simulink model "AFCS_MODEL1"  (R2020b)
settings: Solver=ode4  StartTime=0.0  StopTime=inf  FixedStep=0.005  RelTol=1e-3  EnableMultiTasking=on
values from neighbouring files (symbols this model uses):
  mulh0 = [Lat0;Lon0;Alt0]    [Initial.m]
  routedata_NEH = zeros(3,30)    [Initial.m]
  routeNum = 17    [Initial.m]
libraries: slrealtimeutilitieslib x2, dspnetwork x2, aerolibanimutils x1, simulink x1
settings Model: Creator=Unicorn  LastModifiedBy=chenjiaqing
settings DataIOCC: ReturnWorkspaceOutputs=off
settings OptimizationCC: LifeSpan=inf
settings DebuggingCC: SFUnexpectedBacktrackingDiag=warning  SFNoUnconditionalDefaultTransitionDiag=warning  ArithmeticOperatorsInVariantConditions=warning
settings SFSimCC: SimUseLocalCustomCode=off  CustomCodeUndefinedFunction=UseInterfaceOnly
settings RTWCC: RTWUseLocalCustomCode=off
settings CodeAppCC: StateflowObjectComments=on
settings GRTTargetCC: TargetLangStandard=C89/C90 (ANSI)
settings ConfigComp: CovMetricSettings=dw  CovSaveCumulativeToWorkspaceVar=on  CovSaveSingleToWorkspaceVar=on  CovExternalEMLEnable=off

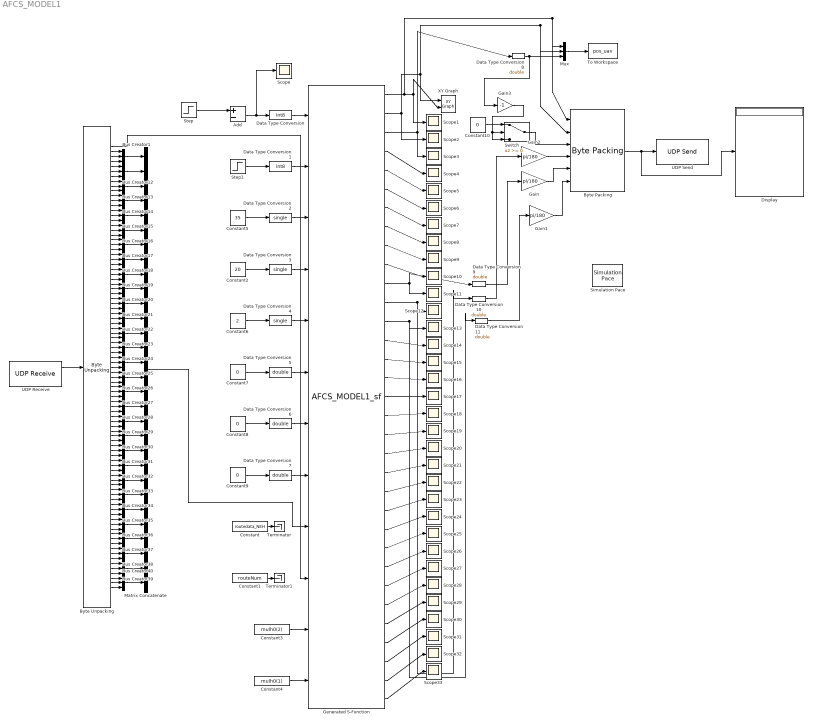
== system AFCS_MODEL1 ==
  Add : Sum  Inputs=+-
  Bus Creator{1,12..40} (30 alike) : BusCreator  Inputs=3
  Byte Packing : slrealtimeutilitieslib/Byte Packing  MaskPackedDataType=double  MaskUnpackedDataTypes={'double','double','double','double','double','double'}  MaskAlignment=8
  Byte Unpacking : slrealtimeutilitieslib/Byte Unpacking  MaskUnpackedDataTypes={'double','double','double','double','double','double','double','double','double','double','double','double','double','double','double','double','double','double','double','double','double','double','double','double','double','double','double','double','double','double','double','double','double','double','double','double','double','double','double','double','double','double','double','double','double','double','double','double','double','double','double','double','double','double','double','double','double','double','double','double','double','double','double','double','double','double','double','double','double','double','double','double','double','double','double','double','double','double','double','double','double','double','double','double','double','double','double','double','double','double','double'}  MaskUnpackedDataSizes={[1],[1],[1],[1],[1],[1],[1],[1],[1],[1],[1],[1],[1],[1],[1],[1],[1],[1],[1],[1],[1],[1],[1],[1],[1],[1],[1],[1],[1],[1],[1],[1],[1],[1],[1],[1],[1],[1],[1],[1],[1],[1],[1],[1],[1],[1],[1],[1],[1],[1],[1],[1],[1],[1],[1],[1],[1],[1],[1],[1],[1],[1],[1],[1],[1],[1],[1],[1],[1],[1],[1],[1],[1],[1],[1],[1],[1],[1],[1],[1],[1],[1],[1],[1],[1],[1],[1],[1],[1],[1],[1]}  MaskAlignment=1
      settings: SourceProductBaseCode=XP
  Constant : Constant  Value=routedata_NEH
  Constant1 : Constant  Value=routeNum
  Constant{7..10} (4 alike) : Constant  Value=0
  Constant2 : Constant  Value=20
  Constant3 : Constant  Value=mulh0(2)
  Constant4 : Constant  Value=mulh0(1)
  Constant5 : Constant  Value=35
  Constant6 : Constant  Value=2
  Data Type Conversion : DataTypeConversion  OutDataTypeStr=int8
  Data Type Conversion1 : DataTypeConversion  OutDataTypeStr=int8
  Data Type Conversion{5..11} (7 alike) : DataTypeConversion  OutDataTypeStr=double
  Data Type Conversion2 : DataTypeConversion  OutDataTypeStr=single
  Data Type Conversion3 : DataTypeConversion  OutDataTypeStr=single
  Data Type Conversion4 : DataTypeConversion  OutDataTypeStr=single
  Display : Display
  Gain : Gain  Gain=pi/180
  Gain1 : Gain  Gain=pi/180
  Gain2 : Gain  Gain=pi/180
  Gain3 : Gain  Gain=-1
  Generated S-Function : S-Function  FunctionName=AFCS_MODEL1_sf  SFunctionModules=""  SFunctionDeploymentMode=off  EnableBusSupport=off  SFcnStateName=DWORK0,DWORK1,DWORK146,DWORK147,DWORK148,DWORK149,DWORK150,DWORK151,DWORK152,DWORK153,DWORK154,DWORK155,DWORK156,DWORK157,DWORK158,DWORK159,DWORK160,DWORK161,DWORK162,DWORK163,DWORK164,DWORK165,DWORK166,DWORK167,DWORK168,DWORK169,DWORK170,DWORK171,DWORK172,DWORK173,DWORK174,DWORK175,DWORK176,DWORK177,DWORK178,DWORK179,DWORK180,DWORK181,DWORK182,DWORK183,DWORK184,DWORK185,DWORK186,DWORK187,DWORK188,DWORK189,DWORK190,DWORK191,DWORK192,DWORK193,DWORK194,DWORK195,DWORK196,DWORK197,DWORK198,DWORK199,DWORK200,DWORK201,DWORK202,DWORK203,DWORK204,DWORK205,DWORK206,DWORK207,DWORK208,DWORK209,DWORK210,DWORK211,DWORK212,DWORK213,DWORK214,DWORK215,DWORK216,DWORK217,DWORK218,DWORK219,DWORK220,DWORK221,DWORK222,DWORK223,DWORK224,DWORK225,DWORK226,DWORK227,DWORK228,DWORK229,DWORK230,DWORK231,DWORK232,DWORK233,DWORK234,DWORK235,DWORK236,DWORK237,DWORK238,DWORK239,DWORK240,DWORK241,DWORK242,DWORK243,DWORK244,DWORK245,DWORK246,DWORK247,DWORK248,DWORK249,DWORK250,DWORK251,DWORK252,DWORK253,DWORK254,DWORK255,DWORK256,DWORK257,DWORK258,DWORK259,DWORK260,DWORK261,DWORK262,DWORK263,DWORK264,DWORK265,DWORK266,DWORK267,DWORK268,DWORK269,DWORK352,DWORK353,DWORK354,DWORK355,DWORK356,DWORK357,DWORK358,DWORK359,DWORK360,DWORK361,DWORK362,DWORK363,DWORK364,DWORK365,DWORK366,DWORK367,DWORK368,DWORK369,DWORK370,DWORK371,DWORK372,DWORK373,DWORK374,DWORK375,DWORK376,DWORK377,DWORK378,DWORK379,DWORK380,DWORK381,DWORK382,DWORK383,DWORK384,DWORK385,DWORK386,DWORK387,DWORK388,DWORK389,DWORK390,DWORK391,DWORK392,DWORK393,DWORK394,DWORK395,DWORK396,DWORK397,DWORK398,DWORK399,DWORK400,DWORK401,DWORK402,DWORK403,DWORK404,DWORK405,DWORK406,DWORK407,DWORK408,DWORK409,DWORK410,DWORK411,DWORK412,DWORK413,DWORK414,DWORK415,DWORK416,DWORK417,DWORK418,DWORK419,DWORK420,DWORK421,DWORK422,DWORK423,DWORK424,DWORK425,DWORK426,DWORK427,DWORK428,DWORK429,DWORK430,DWORK431,DWORK432,DWORK433,DWORK434,DWORK435,DWORK436,DWORK437,DWORK438,DWORK439,DWORK440,DWORK441,DWORK442,DWORK443,DWORK444,DWORK445,DWORK446,DWORK447,DWORK448,DWORK449,DWORK450,DWORK451,DWORK452,DWORK453,DWORK454,DWORK455,DWORK456,DWORK457,DWORK458,DWORK459,DWORK460,DWORK461,DWORK462,DWORK463,DWORK464,DWORK465,DWORK466,DWORK467,DWORK468,DWORK469,DWORK470,DWORK471,DWORK472,DWORK473,DWORK474,DWORK475,DWORK476,DWORK477,DWORK478,DWORK479,DWORK480,DWORK481,DWORK482,DWORK483,DWORK484,DWORK485,DWORK486,DWORK487,DWORK488,DWORK489,DWORK490,DWORK491,DWORK492,DWORK493,DWORK494,DWORK495,DWORK496,DWORK497,DWORK498,DWORK499,DWORK500,DWORK501,DWORK502,DWORK503  mask{rtw_sf_name=AFCS_MODEL1_sf, showVar=off}
      mask prompts: rtw_sf_name "Simulink:masks:GenSFuncName_MP"; showVar "Simulink:masks:GenSFuncShowModuleList_MP"
      mask help: Simulink:masks:GenSFuncDesc_MD
      mask init:
      | displist = '';
      | if ~strcmp(get_param(gcb, 'FunctionName'), rtw_sf_name);
      |   set_param(gcb, 'FunctionName', rtw_sf_name);
      | end
      | % Check if we are generating code
      | rtw_mode = false;
      | if strcmpi(get_param(bdroot(gcb),'SimulationStatus'),'Initializing')
      | 	rtw_mode = strcmpi(get_param(bdroot(gcb),'BuildingRTWCode'),'on') && ...
      | 		~strcmpi(get_param(bdroot(gcb),'TargetStyle'),'SimulationTarget');
      | end
      | if showVar || rtw_mode
      | 	if exist('rtwsfunc') == 2 | exist('rtwsfunc') == 6
      | 		tmplist = rtwsfunc(rtw_sf_name,gcb);
      | 		tmplist = DAStudio.message('Simulink:masks:GenSFuncListOfModules_IC', tmplist);
      | 	elseif showVar
      | 		tmplist1 = DAStudio.message('Simulink:masks:GenSFuncListOfModules_IC', '');
      |         tmplist2 = DAStudio.message('Simulink:masks:GenSFuncNotLicensed_IC');
      |         tmplist = [tmplist1 tmplist2];
      |  	end
      | end
      | if showVar
      |   displist = tmplist;
      | end
      settings: SFcnIsStateOwnerBlock=on
      settings: CopyFcn=|
      | if ~strcmp(get_param(gcb,'Linkstatus'),'none') && ...
      | ~strcmp(get_param(gcb,'Linkstatus'),'implicit')
      |   set_param(gcb,'LinkStatus','none');
      | end
      mask Help: eval('feval(''rtwprivate'',''rtwhelpview'',''rtw_sfcn_block'')');
      mask Display:
      | port_label('input',1,'YD_MODE');
      | port_label('input',2,'AT_MODE');
      | port_label('input',3,'DV');
      | port_label('input',4,'CMD_PhiC');
      | port_label('input',5,'CMD_HdotC');
      | port_label('input',6,'Vx_wind');
      | port_label('input',7,'Vy_wind');
      | port_label('input',8,'Vz_wind');
      | port_label('input',9,'routedata_NEH');
      | port_label('input',10,'piontNum');
      | port_label('input',11,'lon0');
      | port_label('input',12,'lat0');
      | port_label('output',1,'X');
      | port_label('output',2,'Y');
      | port_label('output',3,'Hp');
      | port_label('output',4,'HBC');
      | port_label('output',5,'Hg');
      | port_label('output',6,'Vx');
      | port_label('output',7,'Vy');
      | port_label('output',8,'Vh');
      | port_label('output',9,'Alpha');
      | port_label('output',10,'Beta');
      | port_label('output',11,'Theta');
      | port_label('output',12,'Phi');
      | port_label('output',13,'Psi');
      | port_label('output',14,'TRK');
      | port_label('output',15,'p');
      | port_label('output',16,'q');
      | port_label('output',17,'r');
      | port_label('output',18,'Ax');
      | port_label('output',19,'Ay');
      | port_label('output',20,'Az');
      | port_label('output',21,'PLA_L');
      | port_label('output',22,'PLA_R');
      | port_label('output',23,'N2_L');
      | port_label('output',24,'N2_R');
      | port_label('output',25,'De_L');
      | port_label('output',26,'De_R');
      | port_label('output',27,'Da_L');
      | port_label('output',28,'Da_R');
      | port_label('output',29,'Dr');
      | port_label('output',30,'VIAS');
      | port_label('output',31,'VTAS');
      | port_label('output',32,'VG');
      | port_label('output',33,'Flyphase');
  Matrix Concatenate : Concatenate  NumInputs=30  Mode=Multidimensional array  ConcatenateDimension=2
  Mux : Mux  Inputs=3
  Scope{,1..33} (34 alike) : Scope
  Simulation Pace : aerolibanimutils/Simulation Pace  SimulationPace=1  SleepMode=MATLAB Thread  OutputPaceError=off  SampleTime=-1
  Step : Step  Time=100  After=0  SampleTime=0
  Step1 : Step  Time=60  SampleTime=0
  Switch : Switch
  Terminator : Terminator
  Terminator1 : Terminator
  To Workspace : ToWorkspace  VariableName=pos_uav  SampleTime=-1
  UDP Receive : dspnetwork/UDP Receive  localURL='0.0.0.0'  localPort=udp_receive0  remoteURL='127.0.0.1'  remotePort=-1  recvBufferSize=91  dims=91  signalDatatype=double  isComplex=off  isVarSize=off  showBlockingTime=off  blockingTime=0  sampletime=-1  blockPlatform=[]
  UDP Send : dspnetwork/UDP Send  remoteURL='127.0.0.1'  remotePort=udp_send0  localURL='0.0.0.0'  localPortSource=Automatically determine  localPort=25000  sendBufferSize=1  sampletime=-1  blockPlatform=[]  separateLengthPort=0
  XY Graph : simulink/Sinks/XY Graph  xmin=-3000  xmax=3000  ymin=-500  ymax=3000  st=-1
  wires:
  Constant3/1 -> Generated S-Function/11
  Constant4/1 -> Generated S-Function/12
  Constant2/1 -> Data Type Conversion3/1
  Step1/1 -> Data Type Conversion1/1
  Constant5/1 -> Data Type Conversion2/1
  Constant6/1 -> Data Type Conversion4/1
  Step/1 -> Add/1
  Add/1 -> Scope/1, Data Type Conversion/1
  Constant7/1 -> Data Type Conversion5/1
  Constant8/1 -> Data Type Conversion6/1
  Constant9/1 -> Data Type Conversion7/1
  Generated S-Function/4 -> Scope4/1
  Generated S-Function/5 -> Scope5/1
  Generated S-Function/6 -> Scope6/1
  Generated S-Function/7 -> Scope7/1
  Generated S-Function/8 -> Scope8/1
  Generated S-Function/9 -> Scope9/1
  Generated S-Function/10 -> Scope10/1
  Generated S-Function/11 -> Scope11/1, Data Type Conversion9/1
  Generated S-Function/12 -> Scope12/1, Data Type Conversion10/1
  Generated S-Function/13 -> Scope13/1, Data Type Conversion11/1
  Generated S-Function/14 -> Scope14/1
  Generated S-Function/15 -> Scope15/1
  Generated S-Function/16 -> Scope16/1
  Generated S-Function/17 -> Scope17/1
  Generated S-Function/18 -> Scope18/1
  Generated S-Function/19 -> Scope19/1
  Generated S-Function/20 -> Scope20/1
  Generated S-Function/21 -> Scope21/1
  Generated S-Function/22 -> Scope22/1
  Generated S-Function/23 -> Scope23/1
  Generated S-Function/24 -> Scope24/1
  Generated S-Function/25 -> Scope25/1
  Generated S-Function/26 -> Scope26/1
  Generated S-Function/27 -> Scope27/1
  Generated S-Function/28 -> Scope28/1
  Generated S-Function/29 -> Scope29/1
  Generated S-Function/30 -> Scope30/1
  Generated S-Function/31 -> Scope31/1
  Generated S-Function/32 -> Scope32/1
  Data Type Conversion/1 -> Generated S-Function/1
  Data Type Conversion1/1 -> Generated S-Function/2
  Data Type Conversion2/1 -> Generated S-Function/3
  Data Type Conversion3/1 -> Generated S-Function/4
  Data Type Conversion4/1 -> Generated S-Function/5
  Data Type Conversion5/1 -> Generated S-Function/6
  Data Type Conversion6/1 -> Generated S-Function/7
  Data Type Conversion7/1 -> Generated S-Function/8
  Generated S-Function/33 -> Scope33/1
  Generated S-Function/1 -> Mux/1, Byte Packing/1, XY Graph/2, Scope1/1
  Generated S-Function/2 -> Mux/2, Byte Packing/2, XY Graph/1, Scope2/1
  Generated S-Function/3 -> Data Type Conversion8/1, Scope3/1
  Mux/1 -> To Workspace/1
  Data Type Conversion8/1 -> Mux/3, Gain3/1
  Byte Packing/1 -> Display/1, UDP Send/1
  Data Type Conversion9/1 -> Gain/1
  Data Type Conversion10/1 -> Gain2/1
  Data Type Conversion11/1 -> Gain1/1
  Gain/1 -> Byte Packing/5
  Gain2/1 -> Byte Packing/4
  Gain1/1 -> Byte Packing/6
  UDP Receive/1 -> Byte Unpacking/1
  Bus Creator1/1 -> Matrix Concatenate/1
  Bus Creator12/1 -> Matrix Concatenate/2
  Bus Creator13/1 -> Matrix Concatenate/3
  Bus Creator14/1 -> Matrix Concatenate/4
  Bus Creator15/1 -> Matrix Concatenate/5
  Bus Creator16/1 -> Matrix Concatenate/6
  Bus Creator17/1 -> Matrix Concatenate/7
  Bus Creator18/1 -> Matrix Concatenate/8
  Bus Creator19/1 -> Matrix Concatenate/9
  Bus Creator20/1 -> Matrix Concatenate/10
  Bus Creator21/1 -> Matrix Concatenate/11
  Bus Creator22/1 -> Matrix Concatenate/12
  Bus Creator23/1 -> Matrix Concatenate/13
  Bus Creator24/1 -> Matrix Concatenate/14
  Bus Creator25/1 -> Matrix Concatenate/15
  Bus Creator26/1 -> Matrix Concatenate/16
  Bus Creator27/1 -> Matrix Concatenate/17
  Bus Creator28/1 -> Matrix Concatenate/18
  Bus Creator29/1 -> Matrix Concatenate/19
  Bus Creator30/1 -> Matrix Concatenate/20
  Bus Creator31/1 -> Matrix Concatenate/21
  Bus Creator32/1 -> Matrix Concatenate/22
  Bus Creator33/1 -> Matrix Concatenate/23
  Bus Creator34/1 -> Matrix Concatenate/24
  Bus Creator35/1 -> Matrix Concatenate/25
  Bus Creator36/1 -> Matrix Concatenate/26
  Bus Creator37/1 -> Matrix Concatenate/27
  Bus Creator38/1 -> Matrix Concatenate/28
  Bus Creator39/1 -> Matrix Concatenate/29
  Bus Creator40/1 -> Matrix Concatenate/30
  Gain3/1 -> Switch/3, Switch/2
  Constant10/1 -> Switch/1
  Switch/1 -> Byte Packing/3
  Byte Unpacking/2 -> Bus Creator1/1
  Byte Unpacking/3 -> Bus Creator1/2
  Byte Unpacking/4 -> Bus Creator1/3
  Byte Unpacking/5 -> Bus Creator12/1
  Byte Unpacking/6 -> Bus Creator12/2
  Byte Unpacking/7 -> Bus Creator12/3
  Byte Unpacking/8 -> Bus Creator13/1
  Byte Unpacking/9 -> Bus Creator13/2
  Byte Unpacking/10 -> Bus Creator13/3
  Byte Unpacking/11 -> Bus Creator14/1
  Byte Unpacking/12 -> Bus Creator14/2
  Byte Unpacking/13 -> Bus Creator14/3
  Byte Unpacking/14 -> Bus Creator15/1
  Byte Unpacking/15 -> Bus Creator15/2
  Byte Unpacking/16 -> Bus Creator15/3
  Byte Unpacking/17 -> Bus Creator16/1
  Byte Unpacking/18 -> Bus Creator16/2
  Byte Unpacking/19 -> Bus Creator16/3
  Byte Unpacking/20 -> Bus Creator17/1
  Byte Unpacking/21 -> Bus Creator17/2
  Byte Unpacking/22 -> Bus Creator17/3
  Byte Unpacking/23 -> Bus Creator18/1
  Byte Unpacking/24 -> Bus Creator18/2
  Byte Unpacking/25 -> Bus Creator18/3
  Byte Unpacking/26 -> Bus Creator19/1
  Byte Unpacking/27 -> Bus Creator19/2
  Byte Unpacking/28 -> Bus Creator19/3
  Byte Unpacking/29 -> Bus Creator20/1
  Byte Unpacking/30 -> Bus Creator20/2
  Byte Unpacking/31 -> Bus Creator20/3
  Byte Unpacking/32 -> Bus Creator21/1
  Byte Unpacking/33 -> Bus Creator21/2
  Byte Unpacking/34 -> Bus Creator21/3
  Byte Unpacking/35 -> Bus Creator22/1
  Byte Unpacking/36 -> Bus Creator22/2
  Byte Unpacking/37 -> Bus Creator22/3
  Byte Unpacking/38 -> Bus Creator23/1
  Byte Unpacking/39 -> Bus Creator23/2
  Byte Unpacking/40 -> Bus Creator23/3
  Byte Unpacking/41 -> Bus Creator24/1
  Byte Unpacking/42 -> Bus Creator24/2
  Byte Unpacking/43 -> Bus Creator24/3
  Byte Unpacking/44 -> Bus Creator25/1
  Byte Unpacking/45 -> Bus Creator25/2
  Byte Unpacking/46 -> Bus Creator25/3
  Byte Unpacking/47 -> Bus Creator26/1
  Byte Unpacking/48 -> Bus Creator26/2
  Byte Unpacking/49 -> Bus Creator26/3
  Byte Unpacking/50 -> Bus Creator27/1
  Byte Unpacking/51 -> Bus Creator27/2
  Byte Unpacking/52 -> Bus Creator27/3
  Byte Unpacking/53 -> Bus Creator28/1
  Byte Unpacking/54 -> Bus Creator28/2
  Byte Unpacking/55 -> Bus Creator28/3
  Byte Unpacking/56 -> Bus Creator29/1
  Byte Unpacking/57 -> Bus Creator29/2
  Byte Unpacking/58 -> Bus Creator29/3
  Byte Unpacking/59 -> Bus Creator30/1
  Byte Unpacking/60 -> Bus Creator30/2
  Byte Unpacking/61 -> Bus Creator30/3
  Byte Unpacking/62 -> Bus Creator31/1
  Byte Unpacking/63 -> Bus Creator31/2
  Byte Unpacking/64 -> Bus Creator31/3
  Byte Unpacking/65 -> Bus Creator32/1
  Byte Unpacking/66 -> Bus Creator32/2
  Byte Unpacking/67 -> Bus Creator32/3
  Byte Unpacking/68 -> Bus Creator33/1
  Byte Unpacking/69 -> Bus Creator33/2
  Byte Unpacking/70 -> Bus Creator33/3
  Byte Unpacking/71 -> Bus Creator34/1
  Byte Unpacking/72 -> Bus Creator34/2
  Byte Unpacking/73 -> Bus Creator34/3
  Byte Unpacking/74 -> Bus Creator35/1
  Byte Unpacking/75 -> Bus Creator35/2
  Byte Unpacking/76 -> Bus Creator35/3
  Byte Unpacking/77 -> Bus Creator36/1
  Byte Unpacking/78 -> Bus Creator36/2
  Byte Unpacking/79 -> Bus Creator36/3
  Byte Unpacking/80 -> Bus Creator37/1
  Byte Unpacking/81 -> Bus Creator37/2
  Byte Unpacking/82 -> Bus Creator37/3
  Byte Unpacking/83 -> Bus Creator38/1
  Byte Unpacking/84 -> Bus Creator38/2
  Byte Unpacking/85 -> Bus Creator38/3
  Byte Unpacking/86 -> Bus Creator39/1
  Byte Unpacking/87 -> Bus Creator39/2
  Byte Unpacking/88 -> Bus Creator39/3
  Byte Unpacking/89 -> Bus Creator40/1
  Byte Unpacking/90 -> Bus Creator40/2
  Byte Unpacking/91 -> Bus Creator40/3
  Constant/1 -> Terminator/1
  Constant1/1 -> Terminator1/1
  Byte Unpacking/1 -> Generated S-Function/10
  Matrix Concatenate/1 -> Generated S-Function/9
